simulink model "BasicAudio_Target"  (R2022b)
settings: Solver=FixedStepDiscrete  StartTime=0.0  StopTime=1  RelTol=1e-3  EnableMultiTasking=on
InitFcn:
  | % Initialize model
  | run([ ModelRootName() 'Init.m' ]);
  | 
  | % load library data
  | GainLibrary_data;
  | % Load saved values from partition process
  | TOP_Mask.LoadMapFromFile(bdroot)
model workspace (MAT data in the model file):
  PreampVolumeTable_Idx : Simulink.Signal (value not decoded)
  Range : Simulink.Signal (value not decoded)
  Table_Idx : Simulink.Signal (value not decoded)
undefined symbols (not defined in the file or in its folder): ModelCfg, RgainBusUtil
libraries: TOP x27, HandyTextFile x14, FeaturePath x7, SetDsm x6, RTC x5, AudioStats x3, CapturedConstLib x3, EdgePorts x2, MuteRamperBtc x1, RgainyBtc x1, simulink_need_slupdate x1, dspsrcs4 x1
(part 3 of 5)

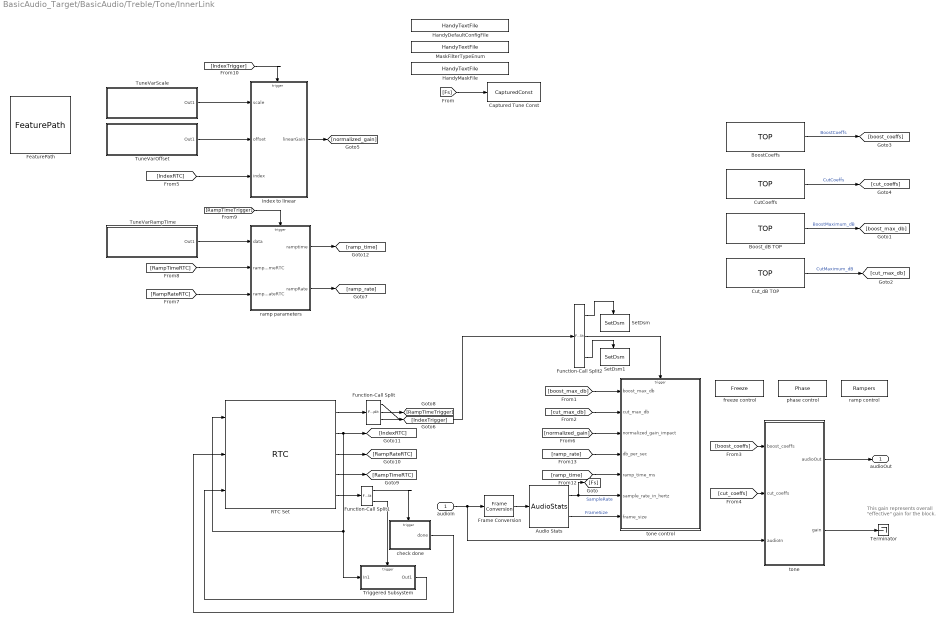
== system BasicAudio_Target/BasicAudio/Treble/Tone/InnerLink ==
  note: This gain represents overall
      | "effective" gain for the block.
  audioIn : Inport
  Audio Stats : AudioStats/AudioStats  DoSampleRate=on  TypeSampleRate=Inherit: auto  DoCallRate=off  TypeCallRate=Inherit: auto  DoFrameSize=on  TypeFrameSize=Inherit: auto  DoChannelCount=off  TypeChannelCount=Inherit: auto  DoTaskRateFactor=off  TypeTaskRateFactor=Inherit: auto  MacroNameRoot=AUDIO  MacroNameRootEval='AUDIO'  IsMacroNameEval=off  MacroSampleRate=off  MacroCallRate=off  MacroFrameSize=off  MacroChannelCount=off  MacroTaskRateFactor=off  MacroTaskId=off  ValidateSampleRate=off  ValueSampleRate=44100  ValidateCallRate=off  ValueCallRate=[]  ValidateFrameSize=off  ValueFrameSize=32  ValidateChannelCount=off  ValueChannelCount=[]  ValidateTaskRateFactor=off  ValueTaskRateFactor=[]
      settings: SourceProductName=Bose Talaria
  BoostCoeffs : TOP/TOP  TriggerInit=[-490 -218 -340 -162]  TopName=BoostCoeffs  DataTypeOut=single  BankNumber=Config.BankNumber  PreOverlay=false  PostOverlay=false  CompatibilityString=[]  Role=Automatic
      settings: SourceProductName=Bose Talaria
  Boost_dB TOP : TOP/TOP  TriggerInit=[-490 -43 -340 13]  TopName=BoostMaximum_dB  DataTypeOut=single  BankNumber=Config.BankNumber  PreOverlay=false  PostOverlay=false  CompatibilityString=[]  Role=Automatic
      settings: SourceProductName=Bose Talaria
  Captured Tune Const : CapturedConstLib/CapturedConst  TriggerInit=[-945 -293 -845 -257]  Role=Automatic
      settings: SourceProductName=Bose Talaria
  CutCoeffs : TOP/TOP  TriggerInit=[-490 -128 -340 -72]  TopName=CutCoeffs  DataTypeOut=single  BankNumber=Config.BankNumber  PreOverlay=false  PostOverlay=false  CompatibilityString=[]  Role=Automatic
      settings: SourceProductName=Bose Talaria
  Cut_dB TOP : TOP/TOP  TriggerInit=[-490 42 -340 98]  TopName=CutMaximum_dB  DataTypeOut=single  BankNumber=Config.BankNumber  PreOverlay=false  PostOverlay=false  CompatibilityString=[]  Role=Automatic
      settings: SourceProductName=Bose Talaria
  FeaturePath : FeaturePath/FeaturePath  FeatureName=Treble  IsGroup=off  GroupNumber=-1  IsModule=off  TriggerInit=[-1855 -266 -1740 -159]
      settings: SourceProductName=Bose Talaria
  Frame Conversion : FrameConversion  OutFrame=Sample-based
  Function-Call Split : FunctionCallSplit  IconShape=distinctive  NumOutputPorts=3
  Function-Call Split1 : FunctionCallSplit  IconShape=distinctive  NumOutputPorts=2  OutputPortLayout=default
  Function-Call Split2 : FunctionCallSplit  IconShape=distinctive  NumOutputPorts=3  OutputPortLayout=default
  HandyDefaultConfigFile : HandyTextFile/HandyTextFile  TemplateSource=Config  FileSuffix=Init  OpenDialogOnLoad=off  UseThisBlockName=off  AddGrandParentNamePrefix=off  TheDefaultText=|  ShowInLibBrowser=on
      | % $(FILENAME) Setup model parameters for each "Init" callback (e.g. update diagram)
      | sample_rate_in_hertz = 44100;
      | frame_size = 32;
      | sysin_channel_count = 2;
      settings: SourceProductName=Bose Talaria
  HandyMaskFile : HandyTextFile/HandyTextFile  TemplateSource=<dialog fields>  FileSuffix=Mask  OpenDialogOnLoad=off  UseThisBlockName=off  AddGrandParentNamePrefix=off  TheDefaultText=|  ShowInLibBrowser=on
      | % $(FILENAME) Setup model parameters for each "Init" callback (e.g. update diagram)
      | sample_rate_in_hertz = 44100;
      | frame_size = 32;
      | sysin_channel_count = 2;
      settings: SourceProductName=Bose Talaria
  MaskFilterTypeEnum : HandyTextFile/HandyTextFile  TemplateSource=Enum  FileSuffix=Init  OpenDialogOnLoad=off  UseThisBlockName=on  AddGrandParentNamePrefix=off  TheDefaultText=|  ShowInLibBrowser=on
      | % $(FILENAME) Setup model parameters for each "Init" callback (e.g. update diagram)
      | sample_rate_in_hertz = 44100;
      | frame_size = 32;
      | sysin_channel_count = 2;
      settings: SourceProductName=Bose Talaria
  RTC Set : RTC/RTC  Description=|  REQ_Priority=RTC_Mask.NormalPriority  RequestAtInit=off  EnableRequest=on  REQElemName1=gain_index  REQElemType1=uint32  REQElemWidth1=1  REQElemInitial1=1  REQElemName2=ramp_db_per_second  REQElemType2=uint32  REQElemWidth2=1  REQElemInitial2=255  REQElemName3=ramp_milliseconds  REQElemType3=uint32  REQElemWidth3=1  REQElemInitial3=0  REQElemType4=uint32  REQElemWidth4=1  REQElemInitial4=[]  REQElemType5=uint32  REQElemWidth5=1  REQElemInitial5=[]  REQElemType6=uint32  REQElemWidth6=1  REQElemInitial6=[]  REQElemType7=uint32  REQElemWidth7=1  REQElemInitial7=[]  REQElemType8=uint32  REQElemWidth8=1  REQElemInitial8=[]  REQElemType9=uint32  REQElemWidth9=1  REQElemInitial9=[]  REQElemType10=uint32  REQElemWidth10=1  REQElemInitial10=[]  EnableResponse=on  EnableRSP_StatusIn=off  RSPElemName1=gain_index  RSPElemType1=uint32  RSPElemWidth1=1  RSPElemType2=uint32  RSPElemWidth2=1  RSPElemType3=uint32  RSPElemWidth3=1  RSPElemType4=uint32  RSPElemWidth4=1  RSPElemType5=uint32  RSPElemWidth5=1  RSPElemType6=uint32  RSPElemWidth6=1  RSPElemType7=uint32  RSPElemWidth7=1  RSPElemType8=uint32  RSPElemWidth8=1  RSPElemType9=uint32  RSPElemWidth9=1  RSPElemType10=uint32  RSPElemWidth10=1  EnableNotification=on  EnableNTF_PrepTrig=off  NTFElemName1=gain_index  NTFElemType1=uint32  NTFElemWidth1=1  NTFElemType2=uint32  NTFElemWidth2=1  NTFElemType3=uint32  NTFElemWidth3=1  NTFElemType4=uint32  NTFElemWidth4=1  NTFElemType5=uint32  NTFElemWidth5=1  NTFElemType6=uint32  NTFElemWidth6=1  NTFElemType7=uint32  NTFElemWidth7=1  NTFElemType8=uint32  NTFElemWidth8=1  NTFElemType9=uint32  NTFElemWidth9=1  NTFElemType10=uint32  NTFElemWidth10=1  MaskMessageName=Set
      | Provide the target value as a 32-bit signed integer index value (to be mapped through a tunable calibration into a normalized float between -1 and 1).
      |  
      | To use slope-based ramping:
      | ----------------------------------
      | When db_per_second has a non-zero value,ramp_milliseconds is ignored and db_per_second controls the ramp.
      |  
      | To use time-based ramping:
      | ----------------------------------
      | The value of db_per_second must be zero for ramp milliseconds to then control the ramping.
      settings: SourceProductName=Bose Talaria
  SetDsm : SetDsm/SetDsm  DataStoreName=Freeze  Value=uint32(1)  SampleTime=-1
      settings: SourceProductName=Bose Talaria
  SetDsm1 : SetDsm/SetDsm  DataStoreName=Freeze  Value=uint32(0)  SampleTime=-1
      settings: SourceProductName=Bose Talaria
  Terminator : Terminator
  Triggered Subsystem : Subsystem  TreatAsAtomicUnit=on
  TuneVarOffset : Subsystem  Description=Offset represents the midpoint of the index range, which separates the 'boost' indices from the 'cut' indices.  mask(Talaria Trivial Tune TOP){TriggerInit=[-1670 -213 -1500 -157], TopName=Offset, DataTypeOut=single, BankNumber=Config.BankNumber, PreOverlay=false, PostOverlay=false, UseSameName=on}
      mask prompts: TriggerInit "Hidden: MoveFcn redraw"; TopName "Name:"; DataTypeOut "Data type:"; BankNumber "Target memory bank number:"; PreOverlay "Requires pre-overlay action:"; PostOverlay "Requires post-overlay action:"; UseSameName "Use same name for tune variable and TOP"
      mask help: The TuneTOP block encapsultes a Target Overlay Parameter, a Tune Variable, and a Trivial Translation between them.
      mask init:
      | [ok,activeTopPath,activeTunePath] = TuneTOP_Mask.Init(gcbh);
      settings: MoveFcn=TuneTOP_Mask.CB_TriggerInit(gcbh);
      mask Callback TriggerInit: TuneTOP_Mask.CB_TriggerInit(gcbh);
      mask TypeOptions TopName: TOP/TopName
      mask TypeOptions DataTypeOut: TOP/DataTypeOut
      mask TypeOptions BankNumber: TOP/BankNumber
      mask TypeOptions PreOverlay: TOP/PreOverlay
      mask TypeOptions PostOverlay: TOP/PostOverlay
      mask Callback UseSameName: TuneTOP_Mask.CB_UseSameName(gcbh);
      mask DialogControl toolPanel Prompt: Tuning Tool Hints
      mask DialogControl DescriptionGroup Prompt: Description
      mask DialogControl DescriptionText Prompt: Offset represents the midpoint of the index range, which separates the 'boost' indices from the 'cut' indices.
      mask DialogControl EditDescription Prompt: Edit Description
      mask DialogControl EditDescription Callback: TuneTOP_Mask.CB_EditDescription(gcbh);
      mask DialogControl TunabilityText Prompt: Easy: Changes nearly every tuning.
      mask DialogControl AdvancedPanel Prompt: Advanced
      mask DialogControl ConvertToFullTranslation Prompt: Irreversible conversion to full translation
      mask DialogControl ConvertToFullTranslation Callback: TuneTOP_Mask.CB_ConvertToFullTranslation(gcbh);
      mask DialogControl ErrorContainer Prompt: Error Messages
      mask Display:
      | % retrieve icon definition
      | [path,w,h] = TuneTOP_Mask.Icon();
      | 
      | % retrieve the block's pixel size
      | pos = get(gcbh,'position');
      | bw = pos(3) - pos(1);
      | bh = pos(4) - pos(2);
      | 
      | % draw centered icon
      | xAdj = bw/2 - w/2 + 5;
      | yAdj = bh/2 - h/2 + 4;
      | for i=1:length(path)
      | 	patch(path(i).x+xAdj, path(i).y+yAdj, path(i).rgb);
      | end
      | 
      | % show the top name or an X
      | if (exist('ok','var') && ok)
      | 	text(bw*0.5, bh*0.2, activeTopPath, 'horizontalAlignment', 'center');
      | 	patch(0,0,[1 1 1]);
      | 	patch(bw,bh,[1 1 1]);
      | else
      | 	tx=bw*0.03;
      | 	ty=bh*0.03;
      | 	patch([0 tx bw bw-tx], [ty 0 bh-ty bh], [1 0 0]);
      | 	patch([0 bw-tx bw tx], [bh-ty 0 ty bh], [1 0 0]);
      | end
  TuneVarRampTime : Subsystem  Description=This is the default ramp time that will be used if the RTC message has a '0' for both ramp time and ramp rate.  mask(Talaria Trivial Tune TOP){TriggerInit=[-1670 -18 -1500 38], TopName=ramptime, DataTypeOut=single, BankNumber=0, PreOverlay=false, PostOverlay=false, UseSameName=on}
      mask prompts: TriggerInit "Hidden: MoveFcn redraw"; TopName "Name:"; DataTypeOut "Data type:"; BankNumber "Target memory bank number:"; PreOverlay "Requires pre-overlay action:"; PostOverlay "Requires post-overlay action:"; UseSameName "Use same name for tune variable and TOP"
      mask help: The TuneTOP block encapsultes a Target Overlay Parameter, a Tune Variable, and a Trivial Translation between them.
      mask init:
      | [ok,activeTopPath,activeTunePath] = TuneTOP_Mask.Init(gcbh);
      settings: MoveFcn=TuneTOP_Mask.CB_TriggerInit(gcbh);
      mask Callback TriggerInit: TuneTOP_Mask.CB_TriggerInit(gcbh);
      mask TypeOptions TopName: TOP/TopName
      mask TypeOptions DataTypeOut: TOP/DataTypeOut
      mask TypeOptions BankNumber: TOP/BankNumber
      mask TypeOptions PreOverlay: TOP/PreOverlay
      mask TypeOptions PostOverlay: TOP/PostOverlay
      mask Callback UseSameName: TuneTOP_Mask.CB_UseSameName(gcbh);
      mask DialogControl toolPanel Prompt: Tuning Tool Hints
      mask DialogControl DescriptionGroup Prompt: Description
      mask DialogControl DescriptionText Prompt: This is the default ramp time that will be used if the RTC message has a '0' for both ramp time and ramp rate.
      mask DialogControl EditDescription Prompt: Edit Description
      mask DialogControl EditDescription Callback: TuneTOP_Mask.CB_EditDescription(gcbh);
      mask DialogControl TunabilityText Prompt: Easy: Changes nearly every tuning.
      mask DialogControl AdvancedPanel Prompt: Advanced
      mask DialogControl ConvertToFullTranslation Prompt: Irreversible conversion to full translation
      mask DialogControl ConvertToFullTranslation Callback: TuneTOP_Mask.CB_ConvertToFullTranslation(gcbh);
      mask DialogControl ErrorContainer Prompt: Error Messages
      mask Display:
      | % retrieve icon definition
      | [path,w,h] = TuneTOP_Mask.Icon();
      | 
      | % retrieve the block's pixel size
      | pos = get(gcbh,'position');
      | bw = pos(3) - pos(1);
      | bh = pos(4) - pos(2);
      | 
      | % draw centered icon
      | xAdj = bw/2 - w/2 + 5;
      | yAdj = bh/2 - h/2 + 4;
      | for i=1:length(path)
      | 	patch(path(i).x+xAdj, path(i).y+yAdj, path(i).rgb);
      | end
      | 
      | % show the top name or an X
      | if (exist('ok','var') && ok)
      | 	text(bw*0.5, bh*0.2, activeTopPath, 'horizontalAlignment', 'center');
      | 	patch(0,0,[1 1 1]);
      | 	patch(bw,bh,[1 1 1]);
      | else
      | 	tx=bw*0.03;
      | 	ty=bh*0.03;
      | 	patch([0 tx bw bw-tx], [ty 0 bh-ty bh], [1 0 0]);
      | 	patch([0 bw-tx bw tx], [bh-ty 0 ty bh], [1 0 0]);
      | end
  TuneVarScale : Subsystem  Description=Scale is used to normalize the linear gain to a value between +/- 1. The range (0,1] represents a boost while the range [-1,0) represents a cut. We use the number of available indices in each range (mapped to gain values between [-1,1]) as the denominator for normalization, i.e. as the 'Scale'.  mask(Talaria Trivial Tune TOP){TriggerInit=[-1670 -283 -1500 -227], TopName=Scale, DataTypeOut=single, BankNumber=Config.BankNumber, PreOverlay=false, PostOverlay=false, UseSameName=on}
      mask prompts: TriggerInit "Hidden: MoveFcn redraw"; TopName "Name:"; DataTypeOut "Data type:"; BankNumber "Target memory bank number:"; PreOverlay "Requires pre-overlay action:"; PostOverlay "Requires post-overlay action:"; UseSameName "Use same name for tune variable and TOP"
      mask help: The TuneTOP block encapsultes a Target Overlay Parameter, a Tune Variable, and a Trivial Translation between them.
      mask init:
      | [ok,activeTopPath,activeTunePath] = TuneTOP_Mask.Init(gcbh);
      settings: MoveFcn=TuneTOP_Mask.CB_TriggerInit(gcbh);
      mask Callback TriggerInit: TuneTOP_Mask.CB_TriggerInit(gcbh);
      mask TypeOptions TopName: TOP/TopName
      mask TypeOptions DataTypeOut: TOP/DataTypeOut
      mask TypeOptions BankNumber: TOP/BankNumber
      mask TypeOptions PreOverlay: TOP/PreOverlay
      mask TypeOptions PostOverlay: TOP/PostOverlay
      mask Callback UseSameName: TuneTOP_Mask.CB_UseSameName(gcbh);
      mask DialogControl toolPanel Prompt: Tuning Tool Hints
      mask DialogControl DescriptionGroup Prompt: Description
      mask DialogControl DescriptionText Prompt: Scale is used to normalize the linear gain to a value between +/- 1. The range (0,1] represents a boost while the range [-1,0) represents a cut. We use the number of available indices in each range (mapped to gain values between [-1,1]) as the denominator for normalization, i.e. as the 'Scale'.
      mask DialogControl EditDescription Prompt: Edit Description
      mask DialogControl EditDescription Callback: TuneTOP_Mask.CB_EditDescription(gcbh);
      mask DialogControl TunabilityText Prompt: Easy: Changes nearly every tuning.
      mask DialogControl AdvancedPanel Prompt: Advanced
      mask DialogControl ConvertToFullTranslation Prompt: Irreversible conversion to full translation
      mask DialogControl ConvertToFullTranslation Callback: TuneTOP_Mask.CB_ConvertToFullTranslation(gcbh);
      mask DialogControl ErrorContainer Prompt: Error Messages
      mask Display:
      | % retrieve icon definition
      | [path,w,h] = TuneTOP_Mask.Icon();
      | 
      | % retrieve the block's pixel size
      | pos = get(gcbh,'position');
      | bw = pos(3) - pos(1);
      | bh = pos(4) - pos(2);
      | 
      | % draw centered icon
      | xAdj = bw/2 - w/2 + 5;
      | yAdj = bh/2 - h/2 + 4;
      | for i=1:length(path)
      | 	patch(path(i).x+xAdj, path(i).y+yAdj, path(i).rgb);
      | end
      | 
      | % show the top name or an X
      | if (exist('ok','var') && ok)
      | 	text(bw*0.5, bh*0.2, activeTopPath, 'horizontalAlignment', 'center');
      | 	patch(0,0,[1 1 1]);
      | 	patch(bw,bh,[1 1 1]);
      | else
      | 	tx=bw*0.03;
      | 	ty=bh*0.03;
      | 	patch([0 tx bw bw-tx], [ty 0 bh-ty bh], [1 0 0]);
      | 	patch([0 bw-tx bw tx], [bh-ty 0 ty bh], [1 0 0]);
      | end
  check done : MATLAB Function  TreatAsAtomicUnit=on
  freeze control : DataStoreMemory  DataStoreName=Freeze  ShowAdditionalParam=off  OutDataTypeStr=uint32
  index to linear : MATLAB Function  TreatAsAtomicUnit=on
  phase control : DataStoreMemory  DataStoreName=Phase  InitialValue=1  ShowAdditionalParam=off  OutDataTypeStr=uint32
  ramp control : DataStoreMemory  DataStoreName=Rampers  InitialValue=Config.DlgRamperInit  ShowAdditionalParam=off  OutDataTypeStr=Bus: rgain_bus
  ramp parameters : MATLAB Function  TreatAsAtomicUnit=on  mask{rampRateBounds=Config.rampRateBounds, rampTimeBounds=Config.rampTimeBounds}
      mask prompts: rampRateBounds "Ramp Rate Bounds"; rampTimeBounds "Ramp Time Bounds"
  tone : MATLAB Function  TreatAsAtomicUnit=on
  tone control : MATLAB Function  TreatAsAtomicUnit=on  mask{rgain_SILENT_GAIN=RgainBusUtil.GetSilentGainLinear}
  audioOut : Outport  VectorParamsAs1DForOutWhenUnconnected=off
  wires:
  Function-Call Split2/1 -> SetDsm/Trigger
  Function-Call Split2/3 -> SetDsm1/Trigger
  Function-Call Split2/2 -> tone control/Trigger
  Triggered Subsystem/1(Out1) -> RTC Set/3
  Function-Call Split1/2 -> Triggered Subsystem/Trigger
  Function-Call Split1/1 -> check done/Trigger
  RTC Set/5 -> Function-Call Split1/1
  TuneVarRampTime/1(Out1) -> ramp parameters/1(data)
  ramp parameters/1(ramptime) -> [ramp_time]
  ramp parameters/2(rampRate) -> [ramp_rate]
  [IndexTrigger] -> index to linear/Trigger
  [RampTimeTrigger] -> ramp parameters/Trigger
  [RampRateRTC] -> ramp parameters/3(rampRateRTC)
  [RampTimeRTC] -> ramp parameters/2(rampTimeRTC)
  [ramp_time] -> tone control/5(ramp_time_ms)
  [ramp_rate] -> tone control/4(db_per_sec)
  [normalized_gain] -> tone control/3(normalized_gain_impact)
  index to linear/1(linearGain) -> [normalized_gain]
  [IndexRTC] -> index to linear/3(index)
  Function-Call Split/2 -> [RampTimeTrigger]
  RTC Set/4 -> [RampTimeRTC]
  RTC Set/3 -> [RampRateRTC]
  RTC Set/2 -> [IndexRTC], Triggered Subsystem/1(In1), RTC Set/1
  TuneVarOffset/1(Out1) -> index to linear/2(offset)
  TuneVarScale/1(Out1) -> index to linear/1(scale)
  tone/1(audioOut) -> audioOut/1
  Function-Call Split/3 -> Function-Call Split2/1
  Audio Stats/2 -> tone control/7(frame_size)  "FrameSize"
  Audio Stats/1 -> [Fs], tone control/6(sample_rate_in_hertz)  "SampleRate"
  Frame Conversion/1 -> Audio Stats/1
  audioIn/1 -> tone/3(audioIn), Frame Conversion/1
  Boost_dB TOP/1 -> [boost_max_db]  "BoostMaximum_dB"
  Cut_dB TOP/1 -> [cut_max_db]  "CutMaximum_dB"
  [boost_max_db] -> tone control/1(boost_max_db)
  [cut_max_db] -> tone control/2(cut_max_db)
  BoostCoeffs/1 -> [boost_coeffs]  "BoostCoeffs"
  CutCoeffs/1 -> [cut_coeffs]  "CutCoeffs"
  [boost_coeffs] -> tone/1(boost_coeffs)
  [cut_coeffs] -> tone/2(cut_coeffs)
  [Fs] -> Captured Tune Const/1
  check done/1(done) -> RTC Set/2
  RTC Set/1 -> Function-Call Split/1
  Function-Call Split/1 -> [IndexTrigger]
  tone/2(gain) -> Terminator/1

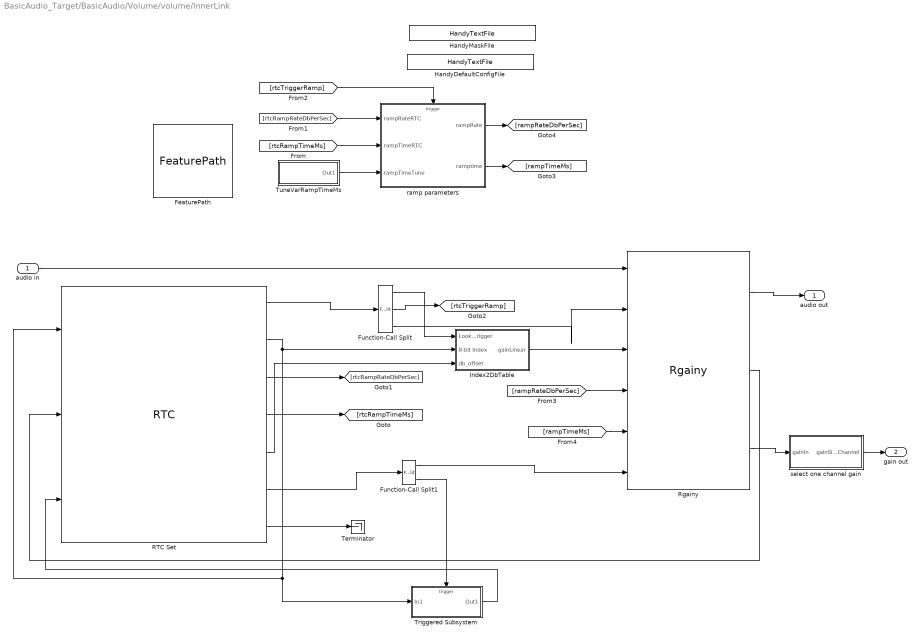
== system BasicAudio_Target/BasicAudio/Volume/volume/InnerLink ==
  audio in : Inport
  FeaturePath : FeaturePath/FeaturePath  FeatureName=Volume  IsGroup=off  GroupNumber=-1  IsModule=off  TriggerInit=[640 269 755 376]
      settings: SourceProductName=Bose Talaria
  Function-Call Split : FunctionCallSplit  IconShape=distinctive  NumOutputPorts=3
  Function-Call Split1 : FunctionCallSplit  IconShape=distinctive  NumOutputPorts=2  OutputPortLayout=default
  HandyDefaultConfigFile : HandyTextFile/HandyTextFile  TemplateSource=Config  FileSuffix=Init  OpenDialogOnLoad=off  UseThisBlockName=off  AddGrandParentNamePrefix=off  TheDefaultText=|  ShowInLibBrowser=on
      | % $(FILENAME) Setup model parameters for each "Init" callback (e.g. update diagram)
      | sample_rate_in_hertz = 44100;
      | frame_size = 32;
      | sysin_channel_count = 2;
      settings: SourceProductName=Bose Talaria
  HandyMaskFile : HandyTextFile/HandyTextFile  TemplateSource=<dialog fields>  FileSuffix=Mask  OpenDialogOnLoad=off  UseThisBlockName=off  AddGrandParentNamePrefix=off  TheDefaultText=|  ShowInLibBrowser=on
      | % $(FILENAME) Setup model parameters for each "Init" callback (e.g. update diagram)
      | sample_rate_in_hertz = 44100;
      | frame_size = 32;
      | sysin_channel_count = 2;
      settings: SourceProductName=Bose Talaria
  Index2DbTable : Subsystem  mask(Blocklib Index2DbTable){Config=Config}
      mask prompts: Config "Index2DbTableConfig"
      mask help: This block contains overlay tuning data for an index-to-dB lookup table. Provide the maximum number of points in the table as a build-time variable. The TuneVar is variable size, but must define at least two points (i.e. two rows, or four values).
      mask init:
      | blkh=gcbh;
      | Config=BTConfig.Assert(blkh,Config);
      | 
      | Config.Validate();
      mask Help:
      | This block contains overlay tuning data which defines an index-to-dB lookup table.
      | Each row of the tuning data contains an index and a dB value.
      | 
      | Tuning data
      | ---------------
      |    tune index: normalized value between 0 and 1
      |    tune value: dB value such as 0 (aka linear "1") or -100 (aka "very quiet")
      | 
      | Inports
      | ----------
      |    trigger: function call trigger that invokes the lookup from inport index to output dB
      |    index: an 8-bit integer index between [0:255] corresponding to the tuning index range [0:1]
      | 
      | Outport
      | -----------
      |    The resulting dB value looked up in the tuned table by using the inbound index
  RTC Set : RTC/RTC  Description=|  REQ_Priority=RTC_Mask.NormalPriority  RequestAtInit=off  EnableRequest=on  REQElemName1=gain_index  REQElemType1=uint32  REQElemWidth1=1  REQElemInitial1=[]  REQElemName2=ramp_db_per_second  REQElemType2=uint32  REQElemWidth2=1  REQElemInitial2=[]  REQElemName3=ramp_milliseconds  REQElemType3=uint32  REQElemWidth3=1  REQElemInitial3=[]  REQElemName4=gain_offset  REQElemType4=int32  REQElemWidth4=1  REQElemInitial4=[]  REQElemType5=uint32  REQElemWidth5=1  REQElemInitial5=[]  REQElemType6=uint32  REQElemWidth6=1  REQElemInitial6=[]  REQElemType7=uint32  REQElemWidth7=1  REQElemInitial7=[]  REQElemType8=uint32  REQElemWidth8=1  REQElemInitial8=[]  REQElemType9=uint32  REQElemWidth9=1  REQElemInitial9=[]  REQElemType10=uint32  REQElemWidth10=1  REQElemInitial10=[]  EnableResponse=on  EnableRSP_StatusIn=off  RSPElemName1=gain_index  RSPElemType1=uint32  RSPElemWidth1=1  RSPElemType2=uint32  RSPElemWidth2=1  RSPElemType3=uint32  RSPElemWidth3=1  RSPElemType4=uint32  RSPElemWidth4=1  RSPElemType5=uint32  RSPElemWidth5=1  RSPElemType6=uint32  RSPElemWidth6=1  RSPElemType7=uint32  RSPElemWidth7=1  RSPElemType8=uint32  RSPElemWidth8=1  RSPElemType9=uint32  RSPElemWidth9=1  RSPElemType10=uint32  RSPElemWidth10=1  EnableNotification=on  EnableNTF_PrepTrig=on  NTFElemName1=gain_index  NTFElemType1=uint32  NTFElemWidth1=1  NTFElemType2=uint32  NTFElemWidth2=1  NTFElemType3=uint32  NTFElemWidth3=1  NTFElemType4=uint32  NTFElemWidth4=1  NTFElemType5=uint32  NTFElemWidth5=1  NTFElemType6=uint32  NTFElemWidth6=1  NTFElemType7=uint32  NTFElemWidth7=1  NTFElemType8=uint32  NTFElemWidth8=1  NTFElemType9=uint32  NTFElemWidth9=1  NTFElemType10=uint32  NTFElemWidth10=1  MaskMessageName=Set
      | Sets new target volume.
      | Provide the target volume as 8 bit index value to be mapped through a tunable VolumeTable.
      |  
      | To use slope-based ramping:
      | ----------------------------------
      | When db_per_second has a non-zero value,ramp_milliseconds is ignored and db_per_second controls the ramp.
      |  
      | To use time-based ramping:
      | ----------------------------------
      | The value of db_per_second must be zero for ramp milliseconds to then control the ramping.
      settings: SourceProductName=Bose Talaria
  Rgainy : RgainyBtc/Rgainy  GainOutEnable=on  Config=Config.Rgainy
      settings: SourceProductName=Bose Blocklib
  Terminator : Terminator
  Triggered Subsystem : Subsystem  TreatAsAtomicUnit=on
  TuneVarRampTimeMs : Subsystem  mask(Talaria Trivial Tune TOP){TriggerInit=[825 324 910 356], TopName=RampTime, DataTypeOut=single, BankNumber=0, PreOverlay=false, PostOverlay=false, UseSameName=on}
      mask prompts: TriggerInit "Hidden: MoveFcn redraw"; TopName "Name:"; DataTypeOut "Data type:"; BankNumber "Target memory bank number:"; PreOverlay "Requires pre-overlay action:"; PostOverlay "Requires post-overlay action:"; UseSameName "Use same name for tune variable and TOP"
      mask help: The TuneTOP block encapsultes a Target Overlay Parameter, a Tune Variable, and a Trivial Translation between them.
      mask init:
      | [ok,activeTopPath,activeTunePath] = TuneTOP_Mask.Init(gcbh);
      settings: MoveFcn=TuneTOP_Mask.CB_TriggerInit(gcbh);
      mask Callback TriggerInit: TuneTOP_Mask.CB_TriggerInit(gcbh);
      mask TypeOptions TopName: TOP/TopName
      mask TypeOptions DataTypeOut: TOP/DataTypeOut
      mask TypeOptions BankNumber: TOP/BankNumber
      mask TypeOptions PreOverlay: TOP/PreOverlay
      mask TypeOptions PostOverlay: TOP/PostOverlay
      mask Callback UseSameName: TuneTOP_Mask.CB_UseSameName(gcbh);
      mask DialogControl toolPanel Prompt: Tuning Tool Hints
      mask DialogControl DescriptionGroup Prompt: Description
      mask DialogControl EditDescription Prompt: Edit Description
      mask DialogControl EditDescription Callback: TuneTOP_Mask.CB_EditDescription(gcbh);
      mask DialogControl TunabilityText Prompt: Easy: Changes nearly every tuning.
      mask DialogControl AdvancedPanel Prompt: Advanced
      mask DialogControl ConvertToFullTranslation Prompt: Irreversible conversion to full translation
      mask DialogControl ConvertToFullTranslation Callback: TuneTOP_Mask.CB_ConvertToFullTranslation(gcbh);
      mask DialogControl ErrorContainer Prompt: Error Messages
      mask Display:
      | % retrieve icon definition
      | [path,w,h] = TuneTOP_Mask.Icon();
      | 
      | % retrieve the block's pixel size
      | pos = get(gcbh,'position');
      | bw = pos(3) - pos(1);
      | bh = pos(4) - pos(2);
      | 
      | % draw centered icon
      | xAdj = bw/2 - w/2 + 5;
      | yAdj = bh/2 - h/2 + 4;
      | for i=1:length(path)
      | 	patch(path(i).x+xAdj, path(i).y+yAdj, path(i).rgb);
      | end
      | 
      | % show the top name or an X
      | if (exist('ok','var') && ok)
      | 	text(bw*0.5, bh*0.2, activeTopPath, 'horizontalAlignment', 'center');
      | 	patch(0,0,[1 1 1]);
      | 	patch(bw,bh,[1 1 1]);
      | else
      | 	tx=bw*0.03;
      | 	ty=bh*0.03;
      | 	patch([0 tx bw bw-tx], [ty 0 bh-ty bh], [1 0 0]);
      | 	patch([0 bw-tx bw tx], [bh-ty 0 ty bh], [1 0 0]);
      | end
  ramp parameters : MATLAB Function  TreatAsAtomicUnit=on
  select one channel gain : MATLAB Function  TreatAsAtomicUnit=on
  audio out : Outport  VectorParamsAs1DForOutWhenUnconnected=off
  gain out : Outport  Port=2
  wires:
  Function-Call Split/1 -> Index2DbTable/1(Lookup Trigger)
  ramp parameters/2(ramptime) -> [rampTimeMs]
  ramp parameters/1(rampRate) -> [rampRateDbPerSec]
  [rtcTriggerRamp] -> ramp parameters/Trigger
  RTC Set/5 -> Index2DbTable/3(db_offset)
  [rampTimeMs] -> Rgainy/5
  RTC Set/4 -> [rtcRampTimeMs]
  [rtcRampRateDbPerSec] -> ramp parameters/1(rampRateRTC)
  Rgainy/2 -> RTC Set/2
  Rgainy/1 -> audio out/1
  audio in/1 -> Rgainy/1
  RTC Set/3 -> [rtcRampRateDbPerSec]
  Function-Call Split1/1 -> Rgainy/6
  Function-Call Split1/2 -> Triggered Subsystem/Trigger
  RTC Set/1 -> Function-Call Split/1
  RTC Set/7 -> Terminator/1
  Function-Call Split/2 -> [rtcTriggerRamp]
  RTC Set/6 -> Function-Call Split1/1
  Function-Call Split/3 -> Rgainy/2
  Index2DbTable/1(gainLinear) -> Rgainy/3
  [rtcRampTimeMs] -> ramp parameters/2(rampTimeRTC)
  TuneVarRampTimeMs/1(Out1) -> ramp parameters/3(rampTimeTune)
  [rampRateDbPerSec] -> Rgainy/4
  select one channel gain/1(gainSingleChannel) -> gain out/1
  Rgainy/3 -> select one channel gain/1(gainIn)
  Triggered Subsystem/1(Out1) -> RTC Set/3
  RTC Set/2 -> Triggered Subsystem/1(In1), RTC Set/1, Index2DbTable/2(8-bit Index)

== system BasicAudio_Target/BasicAudio/Balance/balance/InnerLink/Triggered Subsystem ==
  In1 : Inport
  Trigger : TriggerPort  TriggerType=function-call  VariantControl=Variant
  Out1 : Outport
  wires:
  In1/1 -> Out1/1

== system BasicAudio_Target/BasicAudio/Balance/balance/InnerLink/TuneVarBoostDisable ==
  TOP : TOP/TOP  TriggerInit=[440 20 585 80]  TopName=BoostDisable  DataTypeOut=single  BankNumber=BankNumber  PreOverlay=PreOverlay  PostOverlay=PostOverlay  CompatibilityString=[]  Role=Automatic
      settings: SourceProductName=Bose Talaria
  TrivialTranslation : Subsystem  mask(Talaria Trivial Translation){TriggerInit=[300 28 350 72]}
      mask prompts: TriggerInit "Hidden: MoveFcn redraw"
      mask help: A trivial translator connects to a TuneVar on the input side and to a TOP (Target Overlay Parameter) for output. The translator then simply copies the value from TuneVar to TOP with no changes.
      mask init:
      | TrivialTranslationMask.Init(gcbh);
      settings: MoveFcn=TrivialTranslationMask.CB_TriggerInit(gcbh);
      mask Callback TriggerInit: TrivialTranslationMask.CB_TriggerInit(gcbh);
      mask Display:
      | % retrieve icon definition
      | [path,w,h] = TrivialTranslationMask.Icon();
      | 
      | % retrieve the block's pixel size
      | pos = get(gcbh,'position');
      | bw = pos(3) - pos(1);
      | bh = pos(4) - pos(2);
      | 
      | % draw centered icon
      | xAdj = bw/2 - w/2;
      | yAdj = bh/2 - h/2;
      | for i=1:length(path)
      |    patch(path(i).x+xAdj, path(i).y+yAdj, path(i).rgb);
      | end
      | disp('COPY   ');
  Out1 : Outport  VectorParamsAs1DForOutWhenUnconnected=off
  wires:
  TOP/1 -> Out1/1  "variable"

== system BasicAudio_Target/BasicAudio/Balance/balance/InnerLink/TuneVarOffset ==
  TOP : TOP/TOP  TriggerInit=[440 20 585 80]  TopName=Offset  DataTypeOut=single  BankNumber=BankNumber  PreOverlay=PreOverlay  PostOverlay=PostOverlay  CompatibilityString=[]  Role=Automatic
      settings: SourceProductName=Bose Talaria
  TrivialTranslation : Subsystem  mask(Talaria Trivial Translation){TriggerInit=[300 28 350 72]}
      mask prompts: TriggerInit "Hidden: MoveFcn redraw"
      mask help: A trivial translator connects to a TuneVar on the input side and to a TOP (Target Overlay Parameter) for output. The translator then simply copies the value from TuneVar to TOP with no changes.
      mask init:
      | TrivialTranslationMask.Init(gcbh);
      settings: MoveFcn=TrivialTranslationMask.CB_TriggerInit(gcbh);
      mask Callback TriggerInit: TrivialTranslationMask.CB_TriggerInit(gcbh);
      mask Display:
      | % retrieve icon definition
      | [path,w,h] = TrivialTranslationMask.Icon();
      | 
      | % retrieve the block's pixel size
      | pos = get(gcbh,'position');
      | bw = pos(3) - pos(1);
      | bh = pos(4) - pos(2);
      | 
      | % draw centered icon
      | xAdj = bw/2 - w/2;
      | yAdj = bh/2 - h/2;
      | for i=1:length(path)
      |    patch(path(i).x+xAdj, path(i).y+yAdj, path(i).rgb);
      | end
      | disp('COPY   ');
  Out1 : Outport  VectorParamsAs1DForOutWhenUnconnected=off
  wires:
  TOP/1 -> Out1/1  "variable"

== system BasicAudio_Target/BasicAudio/Balance/balance/InnerLink/TuneVarRampTime ==
  TOP : TOP/TOP  TriggerInit=[440 20 585 80]  TopName=RampTime  DataTypeOut=single  BankNumber=BankNumber  PreOverlay=PreOverlay  PostOverlay=PostOverlay  CompatibilityString=[]  Role=Automatic
      settings: SourceProductName=Bose Talaria
  TrivialTranslation : Subsystem  mask(Talaria Trivial Translation){TriggerInit=[300 28 350 72]}
      mask prompts: TriggerInit "Hidden: MoveFcn redraw"
      mask help: A trivial translator connects to a TuneVar on the input side and to a TOP (Target Overlay Parameter) for output. The translator then simply copies the value from TuneVar to TOP with no changes.
      mask init:
      | TrivialTranslationMask.Init(gcbh);
      settings: MoveFcn=TrivialTranslationMask.CB_TriggerInit(gcbh);
      mask Callback TriggerInit: TrivialTranslationMask.CB_TriggerInit(gcbh);
      mask Display:
      | % retrieve icon definition
      | [path,w,h] = TrivialTranslationMask.Icon();
      | 
      | % retrieve the block's pixel size
      | pos = get(gcbh,'position');
      | bw = pos(3) - pos(1);
      | bh = pos(4) - pos(2);
      | 
      | % draw centered icon
      | xAdj = bw/2 - w/2;
      | yAdj = bh/2 - h/2;
      | for i=1:length(path)
      |    patch(path(i).x+xAdj, path(i).y+yAdj, path(i).rgb);
      | end
      | disp('COPY   ');
  Out1 : Outport  VectorParamsAs1DForOutWhenUnconnected=off
  wires:
  TOP/1 -> Out1/1  "variable"

== system BasicAudio_Target/BasicAudio/Balance/balance/InnerLink/TuneVarSilentBass ==
  TOP : TOP/TOP  TriggerInit=[440 20 585 80]  TopName=SleepingBeautyMutesBass  DataTypeOut=single  BankNumber=BankNumber  PreOverlay=PreOverlay  PostOverlay=PostOverlay  CompatibilityString=[]  Role=Automatic
      settings: SourceProductName=Bose Talaria
  TrivialTranslation : Subsystem  mask(Talaria Trivial Translation){TriggerInit=[300 28 350 72]}
      mask prompts: TriggerInit "Hidden: MoveFcn redraw"
      mask help: A trivial translator connects to a TuneVar on the input side and to a TOP (Target Overlay Parameter) for output. The translator then simply copies the value from TuneVar to TOP with no changes.
      mask init:
      | TrivialTranslationMask.Init(gcbh);
      settings: MoveFcn=TrivialTranslationMask.CB_TriggerInit(gcbh);
      mask Callback TriggerInit: TrivialTranslationMask.CB_TriggerInit(gcbh);
      mask Display:
      | % retrieve icon definition
      | [path,w,h] = TrivialTranslationMask.Icon();
      | 
      | % retrieve the block's pixel size
      | pos = get(gcbh,'position');
      | bw = pos(3) - pos(1);
      | bh = pos(4) - pos(2);
      | 
      | % draw centered icon
      | xAdj = bw/2 - w/2;
      | yAdj = bh/2 - h/2;
      | for i=1:length(path)
      |    patch(path(i).x+xAdj, path(i).y+yAdj, path(i).rgb);
      | end
      | disp('COPY   ');
  Out1 : Outport  VectorParamsAs1DForOutWhenUnconnected=off
  wires:
  TOP/1 -> Out1/1  "variable"

== system BasicAudio_Target/BasicAudio/Balance/balance/InnerLink/TuneVarSilentExtreme ==
  TOP : TOP/TOP  TriggerInit=[440 20 585 80]  TopName=EnableSilentExtreme  DataTypeOut=single  BankNumber=BankNumber  PreOverlay=PreOverlay  PostOverlay=PostOverlay  CompatibilityString=[]  Role=Automatic
      settings: SourceProductName=Bose Talaria
  TrivialTranslation : Subsystem  mask(Talaria Trivial Translation){TriggerInit=[300 28 350 72]}
      mask prompts: TriggerInit "Hidden: MoveFcn redraw"
      mask help: A trivial translator connects to a TuneVar on the input side and to a TOP (Target Overlay Parameter) for output. The translator then simply copies the value from TuneVar to TOP with no changes.
      mask init:
      | TrivialTranslationMask.Init(gcbh);
      settings: MoveFcn=TrivialTranslationMask.CB_TriggerInit(gcbh);
      mask Callback TriggerInit: TrivialTranslationMask.CB_TriggerInit(gcbh);
      mask Display:
      | % retrieve icon definition
      | [path,w,h] = TrivialTranslationMask.Icon();
      | 
      | % retrieve the block's pixel size
      | pos = get(gcbh,'position');
      | bw = pos(3) - pos(1);
      | bh = pos(4) - pos(2);
      | 
      | % draw centered icon
      | xAdj = bw/2 - w/2;
      | yAdj = bh/2 - h/2;
      | for i=1:length(path)
      |    patch(path(i).x+xAdj, path(i).y+yAdj, path(i).rgb);
      | end
      | disp('COPY   ');
  Out1 : Outport  VectorParamsAs1DForOutWhenUnconnected=off
  wires:
  TOP/1 -> Out1/1  "variable"

== system BasicAudio_Target/BasicAudio/Balance/balance/InnerLink/TuneVarTable ==
  TOP_TableIDb : TOP/TOP  TriggerInit=[455 -5 600 35]  TopName=TableDb  DataTypeOut=single  BankNumber=0  PreOverlay=false  PostOverlay=false  CompatibilityString=[]  Role=Automatic
      settings: SourceProductName=Bose Talaria
  TOP_TableIdx : TOP/TOP  TriggerInit=[455 65 600 105]  TopName=TableIdx  DataTypeOut=single  BankNumber=Config.BankNumber  PreOverlay=false  PostOverlay=false  CompatibilityString=[]  Role=Automatic
      settings: SourceProductName=Bose Talaria
  TableDb : Outport  VectorParamsAs1DForOutWhenUnconnected=off
  TableIdx : Outport  Port=2  VectorParamsAs1DForOutWhenUnconnected=off
  wires:
  TOP_TableIDb/1 -> TableDb/1  "TableDb"
  TOP_TableIdx/1 -> TableIdx/1  "TableIdx"

== system BasicAudio_Target/BasicAudio/Bass/Tone/InnerLink/Triggered Subsystem ==
  In1 : Inport
  Trigger : TriggerPort  TriggerType=function-call  VariantControl=Variant
  Out1 : Outport
  wires:
  In1/1 -> Out1/1

== system BasicAudio_Target/BasicAudio/Bass/Tone/InnerLink/TuneVarOffset ==
  TOP : TOP/TOP  TriggerInit=[440 20 585 80]  TopName=Offset  DataTypeOut=single  BankNumber=BankNumber  PreOverlay=PreOverlay  PostOverlay=PostOverlay  CompatibilityString=[]  Role=Automatic
      settings: SourceProductName=Bose Talaria
  TrivialTranslation : Subsystem  mask(Talaria Trivial Translation){TriggerInit=[300 28 350 72]}
      mask prompts: TriggerInit "Hidden: MoveFcn redraw"
      mask help: A trivial translator connects to a TuneVar on the input side and to a TOP (Target Overlay Parameter) for output. The translator then simply copies the value from TuneVar to TOP with no changes.
      mask init:
      | TrivialTranslationMask.Init(gcbh);
      settings: MoveFcn=TrivialTranslationMask.CB_TriggerInit(gcbh);
      mask Callback TriggerInit: TrivialTranslationMask.CB_TriggerInit(gcbh);
      mask Display:
      | % retrieve icon definition
      | [path,w,h] = TrivialTranslationMask.Icon();
      | 
      | % retrieve the block's pixel size
      | pos = get(gcbh,'position');
      | bw = pos(3) - pos(1);
      | bh = pos(4) - pos(2);
      | 
      | % draw centered icon
      | xAdj = bw/2 - w/2;
      | yAdj = bh/2 - h/2;
      | for i=1:length(path)
      |    patch(path(i).x+xAdj, path(i).y+yAdj, path(i).rgb);
      | end
      | disp('COPY   ');
  Out1 : Outport  VectorParamsAs1DForOutWhenUnconnected=off
  wires:
  TOP/1 -> Out1/1  "variable"

== system BasicAudio_Target/BasicAudio/Bass/Tone/InnerLink/TuneVarRampTime ==
  TOP : TOP/TOP  TriggerInit=[440 20 585 80]  TopName=ramptime  DataTypeOut=single  BankNumber=BankNumber  PreOverlay=PreOverlay  PostOverlay=PostOverlay  CompatibilityString=[]  Role=Automatic
      settings: SourceProductName=Bose Talaria
  TrivialTranslation : Subsystem  mask(Talaria Trivial Translation){TriggerInit=[300 28 350 72]}
      mask prompts: TriggerInit "Hidden: MoveFcn redraw"
      mask help: A trivial translator connects to a TuneVar on the input side and to a TOP (Target Overlay Parameter) for output. The translator then simply copies the value from TuneVar to TOP with no changes.
      mask init:
      | TrivialTranslationMask.Init(gcbh);
      settings: MoveFcn=TrivialTranslationMask.CB_TriggerInit(gcbh);
      mask Callback TriggerInit: TrivialTranslationMask.CB_TriggerInit(gcbh);
      mask Display:
      | % retrieve icon definition
      | [path,w,h] = TrivialTranslationMask.Icon();
      | 
      | % retrieve the block's pixel size
      | pos = get(gcbh,'position');
      | bw = pos(3) - pos(1);
      | bh = pos(4) - pos(2);
      | 
      | % draw centered icon
      | xAdj = bw/2 - w/2;
      | yAdj = bh/2 - h/2;
      | for i=1:length(path)
      |    patch(path(i).x+xAdj, path(i).y+yAdj, path(i).rgb);
      | end
      | disp('COPY   ');
  Out1 : Outport  VectorParamsAs1DForOutWhenUnconnected=off
  wires:
  TOP/1 -> Out1/1  "variable"

== system BasicAudio_Target/BasicAudio/Bass/Tone/InnerLink/TuneVarScale ==
  TOP : TOP/TOP  TriggerInit=[440 20 585 80]  TopName=Scale  DataTypeOut=single  BankNumber=BankNumber  PreOverlay=PreOverlay  PostOverlay=PostOverlay  CompatibilityString=[]  Role=Automatic
      settings: SourceProductName=Bose Talaria
  TrivialTranslation : Subsystem  mask(Talaria Trivial Translation){TriggerInit=[300 28 350 72]}
      mask prompts: TriggerInit "Hidden: MoveFcn redraw"
      mask help: A trivial translator connects to a TuneVar on the input side and to a TOP (Target Overlay Parameter) for output. The translator then simply copies the value from TuneVar to TOP with no changes.
      mask init:
      | TrivialTranslationMask.Init(gcbh);
      settings: MoveFcn=TrivialTranslationMask.CB_TriggerInit(gcbh);
      mask Callback TriggerInit: TrivialTranslationMask.CB_TriggerInit(gcbh);
      mask Display:
      | % retrieve icon definition
      | [path,w,h] = TrivialTranslationMask.Icon();
      | 
      | % retrieve the block's pixel size
      | pos = get(gcbh,'position');
      | bw = pos(3) - pos(1);
      | bh = pos(4) - pos(2);
      | 
      | % draw centered icon
      | xAdj = bw/2 - w/2;
      | yAdj = bh/2 - h/2;
      | for i=1:length(path)
      |    patch(path(i).x+xAdj, path(i).y+yAdj, path(i).rgb);
      | end
      | disp('COPY   ');
  Out1 : Outport  VectorParamsAs1DForOutWhenUnconnected=off
  wires:
  TOP/1 -> Out1/1  "variable"

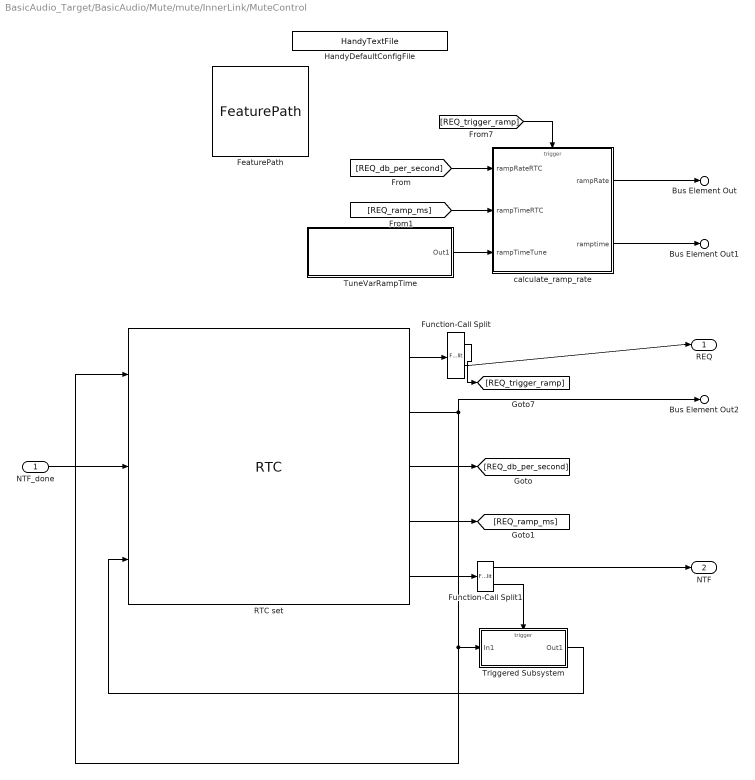
== system BasicAudio_Target/BasicAudio/Mute/mute/InnerLink/MuteControl ==
  NTF_done : Inport
  FeaturePath : FeaturePath/FeaturePath  FeatureName=Mute  IsGroup=off  GroupNumber=-1  IsModule=off  TriggerInit=[180 39 295 146]
      settings: SourceProductName=Bose Talaria
  Function-Call Split : FunctionCallSplit  IconShape=distinctive  NumOutputPorts=2
  Function-Call Split1 : FunctionCallSplit  IconShape=distinctive  NumOutputPorts=2  OutputPortLayout=default
  HandyDefaultConfigFile : HandyTextFile/HandyTextFile  TemplateSource=Config  FileSuffix=Init  OpenDialogOnLoad=off  UseThisBlockName=off  AddGrandParentNamePrefix=off  TheDefaultText=|  ShowInLibBrowser=on
      | % $(FILENAME) Setup model parameters for each "Init" callback (e.g. update diagram)
      | sample_rate_in_hertz = 44100;
      | frame_size = 32;
      | sysin_channel_count = 2;
      settings: SourceProductName=Bose Talaria
  RTC set : RTC/RTC  Description="Command a mute by specifying whether mute is active (non zero mute_switch) or inactive (mute_switch is \"0\"). If db_per_second is non-zero, it commands the timing of the mute, otherwise the ramp_milliseconds is used."  REQ_Priority=RTC_Mask.NormalPriority  RequestAtInit=off  EnableRequest=on  REQElemName1=mute_switch  REQElemType1=uint32  REQElemWidth1=1  REQElemInitial1=[]  REQElemName2=ramp_db_per_second  REQElemType2=uint32  REQElemWidth2=1  REQElemInitial2=[]  REQElemName3=ramp_milliseconds  REQElemType3=uint32  REQElemWidth3=1  REQElemInitial3=[]  REQElemType4=uint32  REQElemWidth4=1  REQElemInitial4=[]  REQElemType5=uint32  REQElemWidth5=1  REQElemInitial5=[]  REQElemType6=uint32  REQElemWidth6=1  REQElemInitial6=[]  REQElemType7=uint32  REQElemWidth7=1  REQElemInitial7=[]  REQElemType8=uint32  REQElemWidth8=1  REQElemInitial8=[]  REQElemType9=uint32  REQElemWidth9=1  REQElemInitial9=[]  REQElemType10=uint32  REQElemWidth10=1  REQElemInitial10=[]  EnableResponse=on  EnableRSP_StatusIn=off  RSPElemName1=mute_switch  RSPElemType1=uint32  RSPElemWidth1=1  RSPElemType2=uint32  RSPElemWidth2=1  RSPElemType3=uint32  RSPElemWidth3=1  RSPElemType4=uint32  RSPElemWidth4=1  RSPElemType5=uint32  RSPElemWidth5=1  RSPElemType6=uint32  RSPElemWidth6=1  RSPElemType7=uint32  RSPElemWidth7=1  RSPElemType8=uint32  RSPElemWidth8=1  RSPElemType9=uint32  RSPElemWidth9=1  RSPElemType10=uint32  RSPElemWidth10=1  EnableNotification=on  EnableNTF_PrepTrig=off  NTFElemName1=mute_switch  NTFElemType1=uint32  NTFElemWidth1=1  NTFElemType2=uint32  NTFElemWidth2=1  NTFElemType3=uint32  NTFElemWidth3=1  NTFElemType4=uint32  NTFElemWidth4=1  NTFElemType5=uint32  NTFElemWidth5=1  NTFElemType6=uint32  NTFElemWidth6=1  NTFElemType7=uint32  NTFElemWidth7=1  NTFElemType8=uint32  NTFElemWidth8=1  NTFElemType9=uint32  NTFElemWidth9=1  NTFElemType10=uint32  NTFElemWidth10=1  MaskMessageName=Set
      settings: SourceProductName=Bose Talaria
  Triggered Subsystem : Subsystem  TreatAsAtomicUnit=on
  TuneVarRampTime : Subsystem  Description=|  mask(Talaria Trivial Tune TOP){TriggerInit=[295 232 465 288], TopName=RampTime, DataTypeOut=single, BankNumber=0, PreOverlay=false, PostOverlay=false, UseSameName=on}
      | Specifies the default value of ramp time for the Mute or Unmute operation.
      | Used only when the RTC message does not contain either ramp rate or ramp time.
      mask prompts: TriggerInit "Hidden: MoveFcn redraw"; TopName "Name:"; DataTypeOut "Data type:"; BankNumber "Target memory bank number:"; PreOverlay "Requires pre-overlay action:"; PostOverlay "Requires post-overlay action:"; UseSameName "Use same name for tune variable and TOP"
      mask help: The TuneTOP block encapsultes a Target Overlay Parameter, a Tune Variable, and a Trivial Translation between them.
      mask init:
      | [ok,activeTopPath,activeTunePath] = TuneTOP_Mask.Init(gcbh);
      settings: MoveFcn=TuneTOP_Mask.CB_TriggerInit(gcbh);
      mask Callback TriggerInit: TuneTOP_Mask.CB_TriggerInit(gcbh);
      mask TypeOptions TopName: TOP/TopName
      mask TypeOptions DataTypeOut: TOP/DataTypeOut
      mask TypeOptions BankNumber: TOP/BankNumber
      mask TypeOptions PreOverlay: TOP/PreOverlay
      mask TypeOptions PostOverlay: TOP/PostOverlay
      mask Callback UseSameName: TuneTOP_Mask.CB_UseSameName(gcbh);
      mask DialogControl toolPanel Prompt: Tuning Tool Hints
      mask DialogControl DescriptionGroup Prompt: Description
      mask DialogControl DescriptionText Prompt:
      | Specifies the default value of ramp time for the Mute or Unmute operation.
      | Used only when the RTC message does not contain either ramp rate or ramp time.
      mask DialogControl EditDescription Prompt: Edit Description
      mask DialogControl EditDescription Callback: TuneTOP_Mask.CB_EditDescription(gcbh);
      mask DialogControl TunabilityText Prompt: Easy: Changes nearly every tuning.
      mask DialogControl AdvancedPanel Prompt: Advanced
      mask DialogControl ConvertToFullTranslation Prompt: Irreversible conversion to full translation
      mask DialogControl ConvertToFullTranslation Callback: TuneTOP_Mask.CB_ConvertToFullTranslation(gcbh);
      mask DialogControl ErrorContainer Prompt: Error Messages
      mask Display:
      | % retrieve icon definition
      | [path,w,h] = TuneTOP_Mask.Icon();
      | 
      | % retrieve the block's pixel size
      | pos = get(gcbh,'position');
      | bw = pos(3) - pos(1);
      | bh = pos(4) - pos(2);
      | 
      | % draw centered icon
      | xAdj = bw/2 - w/2 + 5;
      | yAdj = bh/2 - h/2 + 4;
      | for i=1:length(path)
      | 	patch(path(i).x+xAdj, path(i).y+yAdj, path(i).rgb);
      | end
      | 
      | % show the top name or an X
      | if (exist('ok','var') && ok)
      | 	text(bw*0.5, bh*0.2, activeTopPath, 'horizontalAlignment', 'center');
      | 	patch(0,0,[1 1 1]);
      | 	patch(bw,bh,[1 1 1]);
      | else
      | 	tx=bw*0.03;
      | 	ty=bh*0.03;
      | 	patch([0 tx bw bw-tx], [ty 0 bh-ty bh], [1 0 0]);
      | 	patch([0 bw-tx bw tx], [bh-ty 0 ty bh], [1 0 0]);
      | end
  calculate_ramp_rate : MATLAB Function  TreatAsAtomicUnit=on
  REQ : Outport
  NTF : Outport  Port=2
  Bus Element Out : Outport  Port=3  PortName=OutBus  Element=rampRate
  Bus Element Out1 : Outport  Port=3  PortName=OutBus  Element=rampTime
  Bus Element Out2 : Outport  Port=3  PortName=OutBus  Element=REQ_mute_switch
  wires:
  RTC set/2 -> Bus Element Out2/1, Triggered Subsystem/1(In1), RTC set/1
  [REQ_db_per_second] -> calculate_ramp_rate/1(rampRateRTC)
  Function-Call Split1/1 -> NTF/1
  Function-Call Split1/2 -> Triggered Subsystem/Trigger
  RTC set/5 -> Function-Call Split1/1
  [REQ_trigger_ramp] -> calculate_ramp_rate/Trigger
  Function-Call Split/1 -> [REQ_trigger_ramp]
  RTC set/1 -> Function-Call Split/1
  TuneVarRampTime/1(Out1) -> calculate_ramp_rate/3(rampTimeTune)
  calculate_ramp_rate/1(rampRate) -> Bus Element Out/1
  [REQ_ramp_ms] -> calculate_ramp_rate/2(rampTimeRTC)
  Triggered Subsystem/1(Out1) -> RTC set/3
  RTC set/3 -> [REQ_db_per_second]
  RTC set/4 -> [REQ_ramp_ms]
  NTF_done/1 -> RTC set/2
  calculate_ramp_rate/2(ramptime) -> Bus Element Out1/1
  Function-Call Split/2 -> REQ/1

== system BasicAudio_Target/BasicAudio/Treble/Tone/InnerLink/Triggered Subsystem ==
  In1 : Inport
  Trigger : TriggerPort  TriggerType=function-call  VariantControl=Variant
  Out1 : Outport
  wires:
  In1/1 -> Out1/1
